simulink model "Iteration2_Transformer_PulseOScillator"  (R2015a)
settings: Solver=ode23t  StartTime=0.0  StopTime=1e-3  RelTol=1e-3
libraries: fl_lib x12, nesl_utility x6, elec_lib x5
settings Model: Creator=saifur  LastModifiedBy=saifur
settings SolverCC: SolverResetMethod=Robust
settings DebuggingCC: UnconnectedInputMsg=none  UnconnectedOutputMsg=none  UnconnectedLineMsg=none

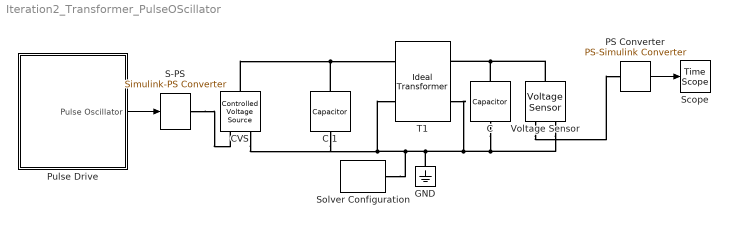
== system Iteration2_Transformer_PulseOScillator ==
  " C " : fl_lib/Electrical/Electrical Elements/Capacitor  c=100e-6 F  r=1e-6 Ohm  g=0 1/Ohm  i_specify=off  i_priority=High  i=0 A  v_specify=off  v_priority=High  v=0 V  vc_specify=off  vc_priority=High  vc=0 V
  " C 1" : fl_lib/Electrical/Electrical Elements/Capacitor  c=100e-6 F  r=1e-6 Ohm  g=0 1/Ohm  i_specify=off  i_priority=High  i=0 A  v_specify=off  v_priority=High  v=0 V  vc_specify=off  vc_priority=High  vc=0 V
  CVS : fl_lib/Electrical/Electrical Sources/Controlled Voltage Source
  GND : fl_lib/Electrical/Electrical Elements/Electrical Reference
  PS Converter : nesl_utility/PS-Simulink Converter  PhysicalDomain=network_engine_domain  SubClassName=ps_output  LeftPortType=input  RightPortType=output  PseudoPeriodic=off  Frequencies=[]  Unit=1  AffineConversion=off
  Pulse Drive : Subsystem
  "S-PS " : nesl_utility/Simulink-PS Converter  PhysicalDomain=network_engine_domain  SubClassName=ps_input  LeftPortType=input  RightPortType=output  PseudoPeriodic=off  Frequencies=[]  NoiseDistribution=none  NoiseParameters=[]  Unit=V  AffineConversion=off  InputFiltering=off  SimscapeFilterOrder=1  InputFilterTimeConstant=0.001  UdotUserProvided=1
  Scope : TimeScope
  Solver Configuration : nesl_utility/Solver Configuration  PhysicalDomain=network_engine_domain  SubClassName=solver  LeftPortType=input  RightPortType=generic  Accelerate=off  Tones=[]  Harmonics=[]  SimulateNoise=off  Profile=off  UseLocalSampling=off  EnableSwitchedLinearOptims=on  FrequencyDomain=off  UseCCode=off  RelTol=0.001  AbsTol=1e-06  MinStep=1e-09  ToWorkspace=off  RevertToSquareIcSolve=off  NumHomotopyIterations=100  DoDC=on  ResidualTolerance=1e-09  UseLocalSolver=off  LocalSolverChoice=NE_BACKWARD_EULER_ADVANCER  LocalSolverSampleTime=0.001  DoFixedCost=off  MaxNonlinIter=3  MaxModeIter=2  LinearAlgebra=Sparse  DelaysMemoryBudget=1024  AutomaticFiltering=on  FilteringTimeConstant=0.001
  T1 : fl_lib/Electrical/Electrical Elements/Ideal Transformer  n=0.05  i1_specify=off  i1_priority=High  i1=0 A  v1_specify=off  v1_priority=High  v1=0 V  i2_specify=off  i2_priority=High  i2=0 A  v2_specify=off  v2_priority=High  v2=0 V
  Voltage Sensor : fl_lib/Electrical/Electrical Sensors/Voltage Sensor
      settings: LogSimulationData=on
  wires:
  PS Converter/1 -> Scope/1
  Pulse Drive/1(Pulse Oscillator) -> "S-PS "/1
  connections:
  " C "/LConn1 -- T1/RConn1 -- Voltage Sensor/LConn1
  " C "/RConn1 -- T1/RConn2 -- GND/LConn1 -- Solver Configuration/RConn1 -- " C 1"/RConn1 -- CVS/RConn2 -- T1/LConn2 -- Voltage Sensor/RConn2
  Voltage Sensor/RConn1 -- PS Converter/LConn1
  CVS/LConn1 -- " C 1"/LConn1 -- T1/LConn1
  "S-PS "/RConn1 -- CVS/RConn1

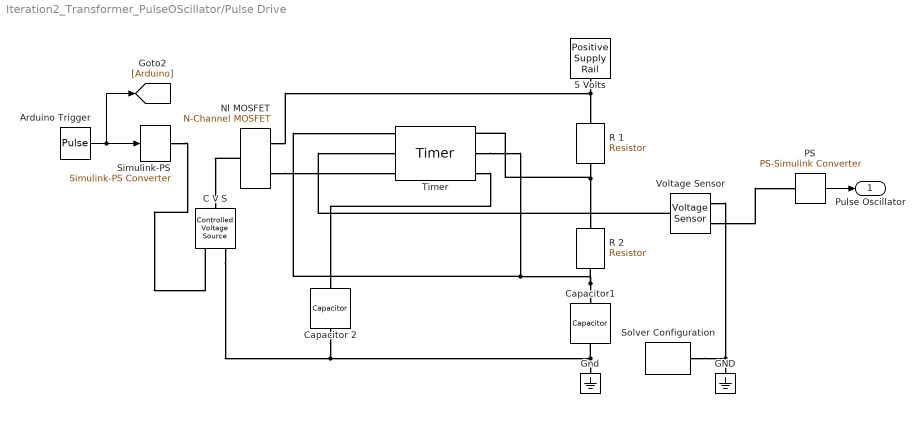
== system Iteration2_Transformer_PulseOScillator/Pulse Drive ==
  5 Volts : elec_lib/Sources/Positive Supply Rail  v0=5 V
  Arduino Trigger : DiscretePulseGenerator  PulseType=Time based  Amplitude=5  Period=0.0001  PulseWidth=50
  C V S : fl_lib/Electrical/Electrical Sources/Controlled Voltage Source
  Capacitor 2 : fl_lib/Electrical/Electrical Elements/Capacitor  c=0.01 uF  r=1e-6 Ohm  g=0 1/Ohm  i_specify=off  i_priority=High  i=0 A  v_specify=off  v_priority=High  v=0 V  vc_specify=off  vc_priority=High  vc=0 V
  Capacitor1 : fl_lib/Electrical/Electrical Elements/Capacitor  c=0.47 nF  r=1e-6 Ohm  g=0 1/Ohm  i_specify=off  i_priority=High  i=0 A  v_specify=off  v_priority=High  v=0 V  vc_specify=off  vc_priority=High  vc=0 V
  GND : fl_lib/Electrical/Electrical Elements/Electrical Reference
  Gnd : fl_lib/Electrical/Electrical Elements/Electrical Reference
  Nl MOSFET : elec_lib/Semiconductor Devices/N-Channel MOSFET  parameterization=1  prmDatasheet=1  prmEquCoeff=1  Beta=5 A/V^2  Rds=0.025 Ohm  Id=6 A  Vgs=10 V  Vth=1.7 V  lam=0 1/V  Tmeas=25 C  RS=1e-4 Ohm  RD=0.01 Ohm  C_param=1  C_GS=270 pF  C_GD=80 pF  C_iss=350 pF  C_rss=80 pF  C_oss=0 pF  C_GS_vec=[ 270 300 290 280 295 255 ] pF  C_GD_vec=[ 450 400 300 190 95 55 ] pF  C_iss_vec=[ 720 700 590 470 390 310 ] pF  C_rss_vec=[ 450 400 300 190 95 55 ] pF  C_oss_vec=[ 900 810 690 420 270 170 ] pF  C_Vds_vec=[ 0.1 0.3 1 3 10 30 ] V  charge_linearity_param=1  C_OX=200 pF  V_C_OX=-0.5 V  dVth_dT=-6 mV/K  Rds_T2=0.037 Ohm  Tmeas2=125 C  BEXDatasheet=-1.5  BEXEquCoeff=-1.5  TdeviceDatasheet=25 C  TdeviceEquCoeff=25 C  Rth=[ 0 10 ] K/W  thermal_mass_parameterization=1  thermal_mass=[ 0 1 ] J/K  thermal_time_constant=[ 0 10 ] s  thermal_mass_initial_temperatures=[ 25 25 ] C
  PS : nesl_utility/PS-Simulink Converter  PhysicalDomain=network_engine_domain  SubClassName=ps_output  LeftPortType=input  RightPortType=output  PseudoPeriodic=off  Frequencies=[]  Unit=1  AffineConversion=off
  R 1 : elec_lib/Passive Devices/Resistor  R=1 kOhm  noise_mode=0  Tdevice=25 C  sample_time=0.001 s  repeatability=1  auto_seed=1503168829  user_seed=0
  R 2 : elec_lib/Passive Devices/Resistor  R=3.5 kOhm  noise_mode=0  Tdevice=25 C  sample_time=0.001 s  repeatability=1  auto_seed=844370171  user_seed=0
  "Simulink-PS " : nesl_utility/Simulink-PS Converter  PhysicalDomain=network_engine_domain  SubClassName=ps_input  LeftPortType=input  RightPortType=output  PseudoPeriodic=off  Frequencies=[]  NoiseDistribution=none  NoiseParameters=[]  Unit=V  AffineConversion=off  InputFiltering=off  SimscapeFilterOrder=1  InputFilterTimeConstant=0.001  UdotUserProvided=1
  Solver Configuration : nesl_utility/Solver Configuration  PhysicalDomain=network_engine_domain  SubClassName=solver  LeftPortType=input  RightPortType=generic  Accelerate=off  Tones=[]  Harmonics=[]  SimulateNoise=off  Profile=off  UseLocalSampling=off  EnableSwitchedLinearOptims=on  FrequencyDomain=off  UseCCode=off  RelTol=0.001  AbsTol=1e-06  MinStep=1e-09  ToWorkspace=off  RevertToSquareIcSolve=off  NumHomotopyIterations=100  DoDC=off  ResidualTolerance=1e-09  UseLocalSolver=off  LocalSolverChoice=NE_TRAPEZOIDAL_ADVANCER  LocalSolverSampleTime=0.001  DoFixedCost=off  MaxNonlinIter=3  MaxModeIter=2  LinearAlgebra=Full  DelaysMemoryBudget=1024  AutomaticFiltering=on  FilteringTimeConstant=0.001
  Timer : elec_lib/Integrated Circuits/Timer  V_CC=5 V  V_OL=0 V  V_OH=5 V  R_OUT=8 Ohm  Delay=1e-7 s  R_DIV=5 kOhm  R_closed=12 Ohm  R_open=5e+8 Ohm
  Voltage Sensor : fl_lib/Electrical/Electrical Sensors/Voltage Sensor
  Pulse Oscillator : Outport
  wires:
  PS/1 -> Pulse Oscillator/1
  Arduino Trigger/1 -> "Simulink-PS "/1, [Arduino]
  connections:
  Timer/RConn2 -- R 2/RConn1 -- Capacitor1/LConn1 -- Timer/LConn1
  Voltage Sensor/RConn1 -- PS/LConn1
  R 1/RConn1 -- Timer/RConn1 -- R 2/LConn1
  Timer/RConn3 -- Capacitor 2/LConn1
  Capacitor 2/RConn1 -- Gnd/LConn1 -- Capacitor1/RConn1 -- C V S/RConn2
  5 Volts/RConn1 -- Nl MOSFET/RConn1 -- R 1/LConn1
  Voltage Sensor/LConn1 -- Timer/LConn2
  Nl MOSFET/LConn1 -- C V S/LConn1
  Nl MOSFET/RConn2 -- Timer/LConn3
  "Simulink-PS "/RConn1 -- C V S/RConn1
  Voltage Sensor/RConn2 -- Solver Configuration/RConn1 -- GND/LConn1
